simulink model "simLab3Generator"  (R2018a)
settings: Solver=ode15s  StartTime=0.0  StopTime=50000  RelTol=1e-3
values from neighbouring files (symbols this model uses):
  area = [A*5+150, B*20+700, C*4+200, D*2+30]    [mainLab3.m]    (also in simulationLab3.m)
  initial_temp_K = TEMP_INSIDE + 273    (= 295)    [simulationLab3.m]
libraries: fl_lib x8, nesl_utility x2
settings Model: Creator=user  LastModifiedBy=user

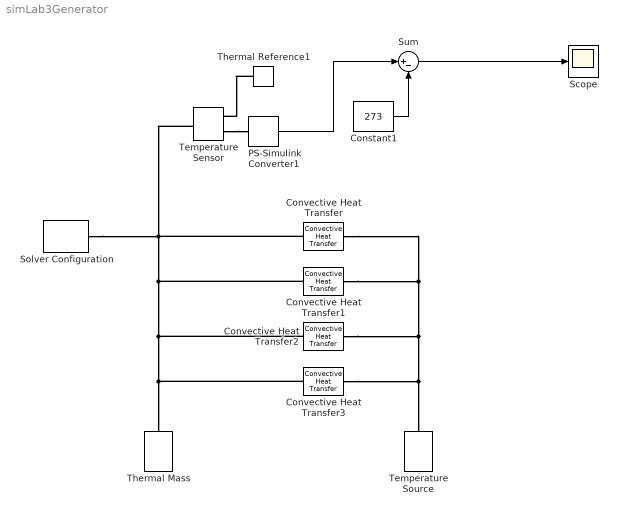
== system simLab3Generator ==
  Constant1 : Constant  Value=273
  Convective Heat Transfer : fl_lib/Thermal/Thermal Elements/Convective Heat Transfer  area=area(1) m^2  heat_tr_coeff=roof_U W/(m^2 * K)  T_specify=off  T_priority=None  T=0 K  T_nominal_specify=off  T_nominal_unit=K  T_nominal_value=1  Q_specify=off  Q_priority=None  Q=0 W  Q_nominal_specify=off  Q_nominal_unit=W  Q_nominal_value=1
  Convective Heat Transfer1 : fl_lib/Thermal/Thermal Elements/Convective Heat Transfer  area=area(2) m^2  heat_tr_coeff=wall_U W/(m^2 * K)  T_specify=off  T_priority=None  T=0 K  T_nominal_specify=off  T_nominal_unit=K  T_nominal_value=1  Q_specify=off  Q_priority=None  Q=0 W  Q_nominal_specify=off  Q_nominal_unit=W  Q_nominal_value=1
  Convective Heat Transfer2 : fl_lib/Thermal/Thermal Elements/Convective Heat Transfer  area=area(3) m^2  heat_tr_coeff=floor_U W/(m^2 * K)  T_specify=off  T_priority=None  T=0 K  T_nominal_specify=off  T_nominal_unit=K  T_nominal_value=1  Q_specify=off  Q_priority=None  Q=0 W  Q_nominal_specify=off  Q_nominal_unit=W  Q_nominal_value=1
  Convective Heat Transfer3 : fl_lib/Thermal/Thermal Elements/Convective Heat Transfer  area=area(4) m^2  heat_tr_coeff=windows_U W/(m^2 * K)  T_specify=off  T_priority=None  T=0 K  T_nominal_specify=off  T_nominal_unit=K  T_nominal_value=1  Q_specify=off  Q_priority=None  Q=0 W  Q_nominal_specify=off  Q_nominal_unit=W  Q_nominal_value=1
  PS-Simulink Converter1 : nesl_utility/PS-Simulink Converter  PhysicalDomain=network_engine_domain  SubClassName=ps_output  LeftPortType=input  RightPortType=output  PseudoPeriodic=off  Frequencies=[]  Unit=K  AffineConversion=off
  Scope : Scope
  Solver Configuration : nesl_utility/Solver Configuration  PhysicalDomain=network_engine_domain  SubClassName=solver  LeftPortType=input  RightPortType=generic  Tones=[]  Harmonics=[]  SimulateNoise=off  Profile=off  UseLocalSampling=off  EnableSwitchedLinearOptims=on  FrequencyDomain=off  UseCCode=off  RelTol=0.001  AbsTol=1e-06  MinStep=1e-09  ToWorkspace=off  RevertToSquareIcSolve=off  NumHomotopyIterations=100  PhasorMode=off  PhasorModeNumHarmonics=1  DoDC=off  ResidualTolerance=1e-09  UseLocalSolver=off  LocalSolverChoice=NE_BACKWARD_EULER_ADVANCER  LocalSolverSampleTime=0.001  DoFixedCost=off  MaxNonlinIter=3  MaxModeIter=2  LinearAlgebra=Sparse  EquationFormulation=NE_TIME_EF  DelaysMemoryBudget=1024  AutomaticFiltering=on  FilteringTimeConstant=0.001
  Sum : Sum  Inputs=|+-
  Temperature Sensor : fl_lib/Thermal/Thermal Sensors/Temperature Sensor
  Temperature Source : fl_lib/Thermal/Thermal Sources/Temperature Source  temperature=outside_temp_K K
      settings: SourceProductName=Simscape
  Thermal Mass : fl_lib/Thermal/Thermal Elements/Thermal Mass  mass=mass_kg kg  sp_heat=HEAT_CAPACITY_unit J/kg/K  T_specify=on  T_priority=High  T=initial_temp_K K  T_nominal_specify=off  T_nominal_unit=K  T_nominal_value=1  Q_specify=off  Q_priority=None  Q=0 W  Q_nominal_specify=off  Q_nominal_unit=W  Q_nominal_value=1
  Thermal Reference1 : fl_lib/Thermal/Thermal Elements/Thermal Reference
  wires:
  Constant1/1 -> Sum/2
  Sum/1 -> Scope/1
  PS-Simulink Converter1/1 -> Sum/1
  connections:
  Convective Heat Transfer/LConn1 -- Temperature Sensor/LConn1 -- Solver Configuration/RConn1 -- Convective Heat Transfer1/LConn1 -- Convective Heat Transfer2/LConn1 -- Convective Heat Transfer3/LConn1 -- Thermal Mass/LConn1
  Convective Heat Transfer/RConn1 -- Convective Heat Transfer1/RConn1 -- Convective Heat Transfer2/RConn1 -- Convective Heat Transfer3/RConn1 -- Temperature Source/LConn1
  Thermal Reference1/LConn1 -- Temperature Sensor/RConn1
  Temperature Sensor/RConn2 -- PS-Simulink Converter1/LConn1
